simulink model "SwitchedPowerRelay_harness"  (Simulink 7.7)
settings: Solver=FixedStepDiscrete  SolverMode=SingleTasking  StartTime=0.0  StopTime=100  FixedStep=srate  RelTol=1e-3
InitFcn:
  | if signalbuilder('SwitchedPowerRelay_harness/Signal_Builder','activegroup') == 7
  |   CD_SWITCHED_POWER_RELAY_DEBOUNCE_NORMAL.DataType = 'uint16';
  |   CD_SWITCHED_POWER_RELAY_DEBOUNCE_NORMAL.Value = 65535;
  | else
  |   CD_SWITCHED_POWER_RELAY_DEBOUNCE_NORMAL.DataType = 'uint16';
  |   CD_SWITCHED_POWER_RELAY_DEBOUNCE_NORMAL.Value = 300;
  | end
  | 
  | if signalbuilder('SwitchedPowerRelay_harness/Signal_Builder','activegroup') == 1
  |   CD_SWITCHED_POWER_RELAY_FUNCTION.DataType = 'uint8';
  |   CD_SWITCHED_POWER_RELAY_FUNCTION.Value = 255;
  | else
  |   CD_SWITCHED_POWER_RELAY_FUNCTION.DataType = 'uint8';
  |   CD_SWITCHED_POWER_RELAY_FUNCTION.Value = 0;
  | end
  | 
  | if signalbuilder('SwitchedPowerRelay_harness/Signal_Builder','activegroup') == 2
  |   CD_SWITCHED_POWER_RELAY_FEEDBACK_FUNCTION.DataType = 'uint8';
  |   CD_SWITCHED_POWER_RELAY_FEEDBACK_FUNCTION.Value = 255;
  | else
  |   CD_SWITCHED_POWER_RELAY_FEEDBACK_FUNCTION.DataType = 'uint8';
  |   CD_SWITCHED_POWER_RELAY_FEEDBACK_FUNCTION.Value = 0;
  | end
undefined symbols (not defined in the file): ACTIVE, CD_SWITCHED_POWER_RELAY_DEBOUNCE_ERROR_ON, CD_SWITCHED_POWER_RELAY_DEBOUNCE_SHUTDOWN, INACTIVE, NON_FUNCTIONAL, OORL, sigbuilder_block, srate, SYS_LIMITED, SYS_POWER_DOWN
libraries: simulink x3, MX_Library x1
Description:
  | Determines state and error condition of the output.
CloseFcn:
  | rtwprivate ssgencode ModelCloseRequest sle_main_controller
settings Model: Creator=smindeman  LastModifiedBy=aliebel  ModifiedComment=smindema -- Wed Nov 01 14:11:02 2006 -- Version 1.321  CovPath=/SLE_Main  CovMetricSettings=dcm  CovHTMLOptions=-aTS=1 -bRG=1 -bTC=1 -hTR=0 -nFC=0 -scm=1 -bcm=1 -xEv=0  covSaveCumulativeToWorkspaceVar=off  CovSaveSingleToWorkspaceVar=off  CovModelRefEnable=off
settings Model: ModifiedHistory=|
  | smindema -- Wed Nov 01 14:11:02 2006 -- Version 1.321
  | 
  | 
  | smindema -- Wed Nov 01 14:09:50 2006 -- Version 1.320
  | added delay on startup to detect error on condition
  | 
  | smindema -- Wed Nov 01 14:09:44 2006 -- Version 1.319
  | 
  | 
  | smindema -- Fri Sep 29 09:20:06 2006 -- Version 1.318
  | updated based on build results
  | 
  | smindema -- Fri Sep 29 09:16:34 2006 -- Version 1.317
  | added open circuit detection
  | 
  | smindema -- Mon Aug 07 10:00:33 2006 -- Version 1.316
  | 
  | 
  | smindema -- Thu Aug 03 10:08:53 2006 -- Version 1.315
  |  removed initialization optimization
  | 
  | smindema -- Thu Jun 08 10:48:55 2006 -- Version 1.314
  | changed optimization settings
  | 
  | smindema -- Thu Apr 20 17:05:53 2006 -- Version 1.313
  | 
  | 
  | smindema -- Thu Apr 20 17:05:12 2006 -- Version 1.311
  | Changed so relay does not turn off with mulitple key.
  | 
  | smindema -- Thu Apr 20 17:05:12 2006 -- Version 1.311
  | Changed so relay does not turn off with mulitple key.
  | 
  | smindema -- Mon Mar 27 16:24:22 2006 -- Version 1.310
  | made dependent on light output.
  | 
  | smindema -- Mon Mar 27 16:13:31 2006 -- Version 1.309
  | 
  | 
  | smindema -- Thu Mar 09 15:09:10 2006 -- Version 1.308
  | made literal lenght max 50
  | 
  | smindema -- Thu Mar 09 14:11:03 2006 -- Version 1.307
  | 
  | 
  | smindema -- Thu Mar 02 09:10:11 2006 -- Version 1.306
  | Made constants mpt parameters.
settings MATStruct: SampleTime=0.01  Offset=0  Priority=[1.0]
settings DataIOCC: LimitDataPoints=off  SaveOutput=off  SaveTime=off
settings OptimizationCC: InlineParams=on  InlineInvariantSignals=on  ExpressionFolding=off  StateBitsets=on  DataBitsets=on  UseTempVars=on  InitFltsAndDblsToZero=on  NoFixptDivByZeroProtection=on  EfficientFloat2IntCast=on
settings DebuggingCC: SaveWithParameterizedLinksMsg=none  SignalResolutionControl=TryResolveAll  MultiTaskDSMMsg=warning  MultiTaskCondExecSysMsg=none  IntegerOverflowMsg=none  ModelReferenceCSMismatchMessage=warning
settings HardwareCC: ProdBitPerInt=16  ProdBitPerPointer=16  ProdIntDivRoundTo=Zero  ProdEndianess=BigEndian  ProdWordSize=16  ProdHWDeviceType=Motorola HC12
settings ModelReferenceCC: ModelReferenceNumInstancesAllowed=Single
settings RTWCC: SystemTargetFile=ert.tlc  GenCodeOnly=on  TemplateMakefile=ert_default_tmf  Description=Real-Time Workshop Embedded Coder (no auto configuration)  GenerateReport=on  RetainRTWFile=on  ProcessScript=ert_make_rtw_hook  IncludeHyperlinkInReport=on  LaunchReport=on  IncludeERTFirstTime=on
settings RTWCC: CustomHeaderCode=|
  | #include "cpp_req_defines.h"
  | #include "cdata.h"
settings CodeAppCC: IgnoreCustomStorageClasses=off  MaxIdLength=50  DefineNamingRule=UpperCase
settings ERTTargetCC: TargetFcnLib=ansi_tfl_tmw.mat  FunctionExecutionProfile=off  MultiwordLength=2048  GenerateSampleERTMain=on  IncludeMdlTerminateFcn=off  SuppressErrorStatus=on  SupportNonFinite=off  SupportComplex=off  PurelyIntegerCode=on  ERTCustomFileTemplate=gen_rtw_req_defines_h.tlc  GlobalDataDefinition=InSeparateSourceFile  GlobalDataReference=InSeparateHeaderFile  ConvertIfToSwitch=off

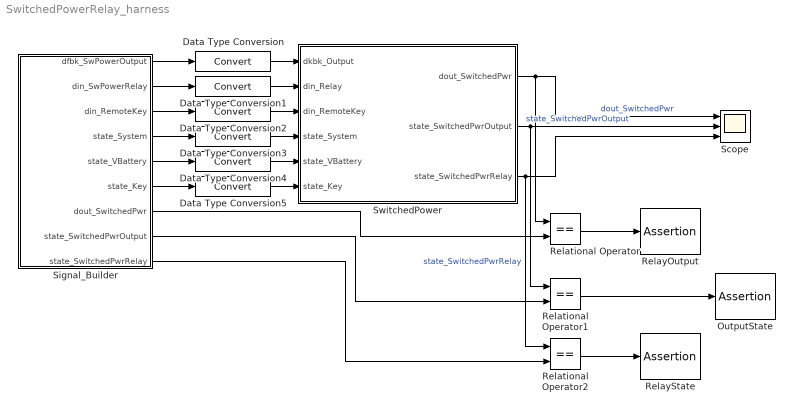
== system SwitchedPowerRelay_harness ==
  Data Type Conversion{,1..5} (6 alike) : DataTypeConversion
  OutputState : Assertion  Enabled=off
  Relational Operator : RelationalOperator  Operator===  OutDataTypeStr=boolean
  Relational Operator1 : RelationalOperator  Operator===  OutDataTypeStr=boolean
  Relational Operator2 : RelationalOperator  Operator===  OutDataTypeStr=boolean
  RelayOutput : Assertion  Enabled=off
  RelayState : Assertion  Enabled=off
  Scope : Scope  NumInputPorts=3
      settings: TimeRange=100  YMin=0~5~7  YMax=1~30~9  MaxDataPoints=50000
  Signal_Builder : Subsystem  Tag=STV Subsys  LoadFcn=sigbuilder_block('load');  StartFcn=sigbuilder_block('start');  StopFcn=sigbuilder_block('stop');  ClipboardFcn=sigbuilder_block('clipboard');  mask(Sigbuilder block){}
      mask help: Sigbuilder GUI
      mask init:
      | if ~strcmp(get_param(bdroot(gcbh),'SimulationStatus'),'stopped') tuvar = sigbuilder_block('maskInit'); end
      settings: CopyFcn=sigbuilder_block('copy');  DeleteFcn=sigbuilder_block('delete');  ModelCloseFcn=sigbuilder_block('modelClose');  PreSaveFcn=sigbuilder_block('preSave');  NameChangeFcn=sigbuilder_block('namechange');  OpenFcn=sigbuilder_block('open',[1510.5 183 1080 624.75 ]);  CloseFcn=sigbuilder_block('close');
      mask Display: plot(0,0,100,100,[10,10,40,40,10],[80,20,20,80,80],[40,10],[50,50], [40,27,10],[65,72,56],[40,25,25,10],[28,28,43,43]);
  SwitchedPower : Subsystem  TreatAsAtomicUnit=on  SystemSampleTime=srate  RTWFileName=mod_Outputs
      settings: RTWSystemCode=Function  RTWFileNameOpts=User specified
  wires:
  Relational Operator/1 -> RelayOutput/1
  Relational Operator1/1 -> OutputState/1
  Relational Operator2/1 -> RelayState/1
  SwitchedPower/1(dout_SwitchedPwr) -> Scope/1, Relational Operator/1  "dout_SwitchedPwr"
  SwitchedPower/2(state_SwitchedPwrOutput) -> Scope/2, Relational Operator1/1  "state_SwitchedPwrOutput"
  SwitchedPower/3(state_SwitchedPwrRelay) -> Scope/3, Relational Operator2/1  "state_SwitchedPwrRelay"
  Signal_Builder/1(dfbk_SwPowerOutput) -> Data Type Conversion/1
  Signal_Builder/2(din_SwPowerRelay) -> Data Type Conversion1/1
  Signal_Builder/3(din_RemoteKey) -> Data Type Conversion2/1
  Signal_Builder/4(state_System) -> Data Type Conversion3/1
  Signal_Builder/5(state_VBattery) -> Data Type Conversion4/1
  Signal_Builder/7(dout_SwitchedPwr) -> Relational Operator/2
  Signal_Builder/8(state_SwitchedPwrOutput) -> Relational Operator1/2
  Signal_Builder/9(state_SwitchedPwrRelay) -> Relational Operator2/2
  Data Type Conversion/1 -> SwitchedPower/1(dkbk_Output)
  Data Type Conversion1/1 -> SwitchedPower/2(din_Relay)
  Data Type Conversion2/1 -> SwitchedPower/3(din_RemoteKey)
  Data Type Conversion3/1 -> SwitchedPower/4(state_System)
  Data Type Conversion4/1 -> SwitchedPower/5(state_VBattery)
  Data Type Conversion5/1 -> SwitchedPower/6(state_Key)
  Signal_Builder/6(state_Key) -> Data Type Conversion5/1

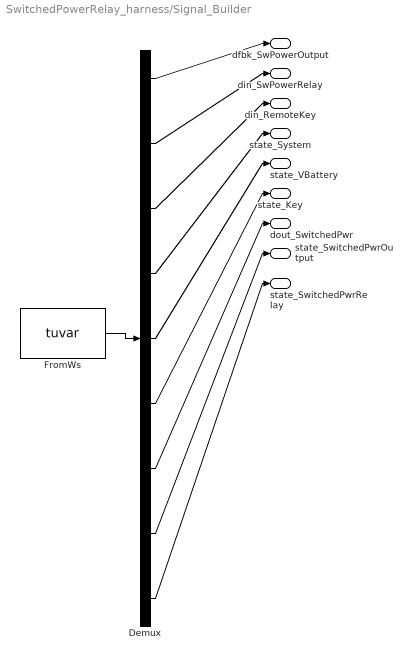
== system SwitchedPowerRelay_harness/Signal_Builder ==
  Demux : Demux  Tag=STV Demux  Outputs=9
  FromWs : FromWorkspace  Tag=STV FromWs  VariableName=tuvar  SampleTime=0  SigBuilderData=DataTag0  VnvData=DataTag1
      SigBuilderData=|
      | common.afterFinalStr = 'Extrapolate'
      | common.sampleTime = 0
      | dataSet(1).timeRange = [0 100]
      | dataSet(1).name = 'T1-Nonfunc'
      | dataSet(2).timeRange = [0 100]
      | dataSet(2).name = 'T2-No_feedback'
      | dataSet(3).timeRange = [0 100]
      | dataSet(3).name = 'T3-NORMAL'
      | dataSet(4).timeRange = [0 100]
      | dataSet(4).name = 'T4-OUT_ERROR'
      | dataSet(5).timeRange = [0 100]
      | dataSet(5).name = 'T5-RELAY_ERROR'
      | dataSet(6).timeRange = [0 100]
      | dataSet(6).name = 'T6-OC_FAILURE'
      | dataSet(7).timeRange = [0 100]
      | dataSet(7).name = 'T7-ERR_UNLIMITED'
      | sbobj.Groups(1).Name = 'T1-Nonfunc'
      | sbobj.Groups(1).Signals(1).Name = 'dfbk_SwPowerOutput'
      | sbobj.Groups(1).Signals(1).XData = [0 40.6 100]
      | sbobj.Groups(1).Signals(1).YData = [0 0 0]
      | sbobj.Groups(1).Signals(2).Name = 'din_SwPowerRelay'
      | sbobj.Groups(1).Signals(2).XData = [0 40.6 100]
      | sbobj.Groups(1).Signals(2).YData = [0 0 0]
      | sbobj.Groups(1).Signals(3).Name = 'din_RemoteKey'
      | sbobj.Groups(1).Signals(3).XData = [0 100]
      | sbobj.Groups(1).Signals(3).YData = [8 8]
      | sbobj.Groups(1).Signals(4).Name = 'state_System'
      | sbobj.Groups(1).Signals(4).XData = [0 40 40 100]
      | sbobj.Groups(1).Signals(4).YData = [0 0 1 1]
      | sbobj.Groups(1).Signals(5).Name = 'state_VBattery'
      | sbobj.Groups(1).Signals(5).XData = [0 100]
      | sbobj.Groups(1).Signals(5).YData = [8 8]
      | sbobj.Groups(1).Signals(6).Name = 'state_Key'
      | sbobj.Groups(1).Signals(6).XData = [0 100]
      | sbobj.Groups(1).Signals(6).YData = [0 0]
      | sbobj.Groups(1).Signals(7).Name = 'dout_SwitchedPwr'
      | sbobj.Groups(1).Signals(7).XData = [0 40.6 100]
      | sbobj.Groups(1).Signals(7).YData = [0 0 0]
      | sbobj.Groups(1).Signals(8).Name = 'state_SwitchedPwrOutput'
      | sbobj.Groups(1).Signals(8).XData = [0 100]
      | sbobj.Groups(1).Signals(8).YData = [8 8]
      | sbobj.Groups(1).Signals(9).Name = 'state_SwitchedPwrRelay'
      | sbobj.Groups(1).Signals(9).XData = [0 100]
      | sbobj.Groups(1).Signals(9).YData = [8 8]
      | sbobj.Groups(2).Name = 'T2-No_feedback'
      | sbobj.Groups(2).Signals(1).Name = 'dfbk_SwPowerOutput'
      | sbobj.Groups(2).Signals(1).XData = [0 40.6 100]
      | sbobj.Groups(2).Signals(1).YData = [0 0 0]
      | sbobj.Groups(2).Signals(2).Name = 'din_SwPowerRelay'
      | sbobj.Groups(2).Signals(2).XData = [0 40.6 100]
      | sbobj.Groups(2).Signals(2).YData = [0 0 0]
      | sbobj.Groups(2).Signals(3).Name = 'din_RemoteKey'
      | sbobj.Groups(2).Signals(3).XData = [0 100]
      | sbobj.Groups(2).Signals(3).YData = [0 0]
      | sbobj.Groups(2).Signals(4).Name = 'state_System'
      | sbobj.Groups(2).Signals(4).XData = [0 10 10 100]
      | sbobj.Groups(2).Signals(4).YData = [0 0 1 1]
      | sbobj.Groups(2).Signals(5).Name = 'state_VBattery'
      | sbobj.Groups(2).Signals(5).XData = [0 62.3 62.3 64.8 64.8 100]
      | sbobj.Groups(2).Signals(5).YData = [8 8 22 22 8 8]
      | sbobj.Groups(2).Signals(6).Name = 'state_Key'
      | sbobj.Groups(2).Signals(6).XData = [0 40.4 40.4 100]
      | sbobj.Groups(2).Signals(6).YData = [0 0 1 1]
      | sbobj.Groups(2).Signals(7).Name = 'dout_SwitchedPwr'
      | sbobj.Groups(2).Signals(7).XData = [0 40.46 40.46 100]
      | sbobj.Groups(2).Signals(7).YData = [0 0 1 1]
      | sbobj.Groups(2).Signals(8).Name = 'state_SwitchedPwrOutput'
      | sbobj.Groups(2).Signals(8).XData = [0 100]
      | sbobj.Groups(2).Signals(8).YData = [8 8]
      | sbobj.Groups(2).Signals(9).Name = 'state_SwitchedPwrRelay'
      | sbobj.Groups(2).Signals(9).XData = [0 100]
      | sbobj.Groups(2).Signals(9).YData = [8 8]
      | sbobj.Groups(3).Name = 'T3-NORMAL'
      | sbobj.Groups(3).Signals(1).Name = 'dfbk_SwPowerOutput'
      | sbobj.Groups(3).Signals(1).XData = [0 10.06 10.06 20 20 30 30 40 40 50 50 60 60 70.06 70.06 75.21 75.21 100]
      | sbobj.Groups(3).Signals(1).YData = [0 0 1 1 0 0 1 1 0 0 1 1 0 0 1 1 0 0]
      | sbobj.Groups(3).Signals(2).Name = 'din_SwPowerRelay'
      | sbobj.Groups(3).Signals(2).XData = [0 10.07 10.07 20 20 30 30 40 40 50 50 60 60 70.07 70.07 75.22 75.22 100]
      | sbobj.Groups(3).Signals(2).YData = [0 0 1 1 0 0 1 1 0 0 1 1 0 0 1 1 0 0]
      | sbobj.Groups(3).Signals(3).Name = 'din_RemoteKey'
      | sbobj.Groups(3).Signals(3).XData = [0 30 30 40 40 50 50 60 60 66.1 66.1 67.3 67.3 100]
      | sbobj.Groups(3).Signals(3).YData = [0 0 1 1 0 0 1 1 0 0 1 1 0 0]
      | sbobj.Groups(3).Signals(4).Name = 'state_System'
      | sbobj.Groups(3).Signals(4).XData = [0 10.7 10.7 20 20 21.5 21.5 30.5 30.5 40 40 41.4 41.4 50.4 50.4 60 60 68.6 68.6 75 75 78.7 78.7 100]
      | sbobj.Groups(3).Signals(4).YData = [0 0 1 1 5 5 0 0 1 1 5 5 0 0 1 1 5 5 0 0 3 3 0 0]
      | sbobj.Groups(3).Signals(5).Name = 'state_VBattery'
      | sbobj.Groups(3).Signals(5).XData = [0 100]
      | sbobj.Groups(3).Signals(5).YData = [8 8]
      | sbobj.Groups(3).Signals(6).Name = 'state_Key'
      | sbobj.Groups(3).Signals(6).XData = [0 10 10 20 20 50 50 60 60 64.3 64.3 65.1 65.1 70 70 75.01 75.01 100]
      | sbobj.Groups(3).Signals(6).YData = [0 0 1 1 0 0 1 1 0 0 1 1 0 0 1 1 0 0]
      | sbobj.Groups(3).Signals(7).Name = 'dout_SwitchedPwr'
      | sbobj.Groups(3).Signals(7).XData = [0 10.05 10.05 20.21 20.21 30 30 40.21 40.21 50 50 60.21 60.21 70.05 70.05 75.22 75.22 100]
      | sbobj.Groups(3).Signals(7).YData = [0 0 1 1 0 0 1 1 0 0 1 1 0 0 1 1 0 0]
      | sbobj.Groups(3).Signals(8).Name = 'state_SwitchedPwrOutput'
      | sbobj.Groups(3).Signals(8).XData = [0 100]
      | sbobj.Groups(3).Signals(8).YData = [8 8]
      | sbobj.Groups(3).Signals(9).Name = 'state_SwitchedPwrRelay'
      | sbobj.Groups(3).Signals(9).XData = [0 100]
      | sbobj.Groups(3).Signals(9).YData = [8 8]
      | sbobj.Groups(4).Name = 'T4-OUT_ERROR'
      | sbobj.Groups(4).Signals(1).Name = 'dfbk_SwPowerOutput'
      | sbobj.Groups(4).Signals(1).XData = [0 5.6 19.8 22.8 30 30 30.03 30.03 41.6 41.6 45 45 45.02 45.02 50.1 50.1 50.22 50.22 58.7 58.7 58.9 58.9 84.3 84.3 85 85 100]
      | sbobj.Groups(4).Signals(1).YData = [1 1 1 1 1 0 0 1 1 0 0 1 1 0 0 1 1 0 0 1 1 0 0 1 1 0 0]
      | sbobj.Groups(4).Signals(2).Name = 'din_SwPowerRelay'
      | sbobj.Groups(4).Signals(2).XData = [0 13.5 13.5 13.51 13.51 30 30 30.03 30.03 41.6 41.6 45 45 45.02 45.02 100]
      | sbobj.Groups(4).Signals(2).YData = [1 1 0 0 1 1 0 0 1 1 0 0 1 1 0 0]
      | sbobj.Groups(4).Signals(3).Name = 'din_RemoteKey'
      | sbobj.Groups(4).Signals(3).XData = [0 50 50 70.1 70.1 100]
      | sbobj.Groups(4).Signals(3).YData = [0 0 1 1 0 0]
      | sbobj.Groups(4).Signals(4).Name = 'state_System'
      | sbobj.Groups(4).Signals(4).XData = [0 20.4 20.4 40 40 41.6 41.6 50 50 70.1 70.1 72.3 72.3 84.3 84.3 84.8 84.8 100]
      | sbobj.Groups(4).Signals(4).YData = [0 0 1 1 5 5 0 0 1 1 5 5 0 0 3 3 0 0]
      | sbobj.Groups(4).Signals(5).Name = 'state_VBattery'
      | sbobj.Groups(4).Signals(5).XData = [0 100]
      | sbobj.Groups(4).Signals(5).YData = [8 8]
      | sbobj.Groups(4).Signals(6).Name = 'state_Key'
      | sbobj.Groups(4).Signals(6).XData = [0 20 20 40 40 80.1 80.1 81.4 81.4 100]
      | sbobj.Groups(4).Signals(6).YData = [0 0 1 1 0 0 1 1 0 0]
      | sbobj.Groups(4).Signals(7).Name = 'dout_SwitchedPwr'
      | sbobj.Groups(4).Signals(7).XData = [0 20.05 20.05 40.21 40.21 50 50 70.31 70.31 80.15 80.15 84.52 84.52 100]
      | sbobj.Groups(4).Signals(7).YData = [0 0 1 1 0 0 1 1 0 0 1 1 0 0]
      | sbobj.Groups(4).Signals(8).Name = 'state_SwitchedPwrOutput'
      | sbobj.Groups(4).Signals(8).XData = [0 0.04 0.04 23.06 23.06 50.53 50.53 70.1 70.1 80.46 80.46 84.83 84.83 88.01 88.01 100]
      | sbobj.Groups(4).Signals(8).YData = [8 8 2 2 8 8 3 3 8 8 3 3 7 7 8 8]
      | sbobj.Groups(4).Signals(9).Name = 'state_SwitchedPwrRelay'
      | sbobj.Groups(4).Signals(9).XData = [0 100]
      | sbobj.Groups(4).Signals(9).YData = [8 8]
      | sbobj.Groups(5).Name = 'T5-RELAY_ERROR'
      | sbobj.Groups(5).Signals(1).Name = 'dfbk_SwPowerOutput'
      | sbobj.Groups(5).Signals(1).XData = [0 5.5 5.5 5.52 5.52 10.7 10.7 21.9 21.9 22.1 22.1 42.7 42.7 44 44.01 50 50 62.1 62.1 62.2 62.2 91 91 100]
      | sbobj.Groups(5).Signals(1).YData = [0 0 1 1 0 0 1 1 0 0 1 1 0 0 0 0 0.98 0.98 0 0 0.98 0.98 0 0]
      | sbobj.Groups(5).Signals(2).Name = 'din_SwPowerRelay'
      | sbobj.Groups(5).Signals(2).XData = [0 42.8 42.8 45 45 45.01 45.01 100]
      | sbobj.Groups(5).Signals(2).YData = [1 1 0 0 1 1 0 0]
      | sbobj.Groups(5).Signals(3).Name = 'din_RemoteKey'
      | sbobj.Groups(5).Signals(3).XData = [0 50 50 90.9 90.9 100]
      | sbobj.Groups(5).Signals(3).YData = [0 0 1 1 0 0]
      | sbobj.Groups(5).Signals(4).Name = 'state_System'
      | sbobj.Groups(5).Signals(4).XData = [0 10 10 42 42 43.7 43.7 50 50 91.7 91.7 94.5 94.5 100]
      | sbobj.Groups(5).Signals(4).YData = [0 0 1 1 5 5 0 0 1 1 5 5 0 0]
      | sbobj.Groups(5).Signals(5).Name = 'state_VBattery'
      | sbobj.Groups(5).Signals(5).XData = [0 100]
      | sbobj.Groups(5).Signals(5).YData = [8 8]
      | sbobj.Groups(5).Signals(6).Name = 'state_Key'
      | sbobj.Groups(5).Signals(6).XData = [0 10 10 41.5 41.5 100]
      | sbobj.Groups(5).Signals(6).YData = [0 0 1 1 0 0]
      | sbobj.Groups(5).Signals(7).Name = 'dout_SwitchedPwr'
      | sbobj.Groups(5).Signals(7).XData = [0 10.05 10.05 42.21 42.21 50 50 91.91 91.91 100]
      | sbobj.Groups(5).Signals(7).YData = [0 0 1 1 0 0 1 1 0 0]
      | sbobj.Groups(5).Signals(8).Name = 'state_SwitchedPwrOutput'
      | sbobj.Groups(5).Signals(8).XData = [0 100]
      | sbobj.Groups(5).Signals(8).YData = [8 8]
      | sbobj.Groups(5).Signals(9).Name = 'state_SwitchedPwrRelay'
      | sbobj.Groups(5).Signals(9).XData = [0 0.04 0.04 13.06 13.06 50.31 50.31 91.7 91.7 100]
      | sbobj.Groups(5).Signals(9).YData = [8 8 2 2 8 8 3 3 8 8]
      | sbobj.Groups(6).Name = 'T6-OC_FAILURE'
      | sbobj.Groups(6).Signals(1).Name = 'dfbk_SwPowerOutput'
      | sbobj.Groups(6).Signals(1).XData = [0 1.03 1.03 1.06 1.06 14 14 14.05 14.05 40 40 50.1 50.1 50.2 50.2 50.3 50.3 54.9 54.9 62.8 62.8 100]
      | sbobj.Groups(6).Signals(1).YData = [0 0 1 1 0 0 1 1 0 0 1 1 0 0 1 1 0 0 1 1 0 0]
      | sbobj.Groups(6).Signals(2).Name = 'din_SwPowerRelay'
      | sbobj.Groups(6).Signals(2).XData = [0 1.03 1.03 18.1 18.1 18.15 18.15 19.9 19.9 55.08 55.08 57.43 57.43 61 61 61.7 61.7 100]
      | sbobj.Groups(6).Signals(2).YData = [0 0 1 1 0 0 1 1 0 0 1 1 0 0 1 1 0 0]
      | sbobj.Groups(6).Signals(3).Name = 'din_RemoteKey'
      | sbobj.Groups(6).Signals(3).XData = [0 100]
      | sbobj.Groups(6).Signals(3).YData = [0 0]
      | sbobj.Groups(6).Signals(4).Name = 'state_System'
      | sbobj.Groups(6).Signals(4).XData = [0 1.5 1.5 19.9 19.9 22.1 22.1 57.2 57.2 58.6 58.6 100]
      | sbobj.Groups(6).Signals(4).YData = [0 0 1 1 5 5 0 0 5 5 0 0]
      | sbobj.Groups(6).Signals(5).Name = 'state_VBattery'
      | sbobj.Groups(6).Signals(5).XData = [0 100]
      | sbobj.Groups(6).Signals(5).YData = [8 8]
      | sbobj.Groups(6).Signals(6).Name = 'state_Key'
      | sbobj.Groups(6).Signals(6).XData = [0 1 1 20 20 55 55 57.2 57.2 100]
      | sbobj.Groups(6).Signals(6).YData = [0 0 1 1 0 0 1 1 0 0]
      | sbobj.Groups(6).Signals(7).Name = 'dout_SwitchedPwr'
      | sbobj.Groups(6).Signals(7).XData = [0 1.05 1.05 20.11 20.11 55.05 55.05 57.41 57.41 100]
      | sbobj.Groups(6).Signals(7).YData = [0 0 1 1 0 0 1 1 0 0]
      | sbobj.Groups(6).Signals(8).Name = 'state_SwitchedPwrOutput'
      | sbobj.Groups(6).Signals(8).XData = [0 1.37 1.37 19.9 19.9 40.31 40.31 53.31 53.31 58.91 58.91 61.04 61.04 62.02 62.02 65.81 65.81 100]
      | sbobj.Groups(6).Signals(8).YData = [8 8 28 28 8 8 7 7 8 8 7 7 2 2 7 7 8 8]
      | sbobj.Groups(6).Signals(9).Name = 'state_SwitchedPwrRelay'
      | sbobj.Groups(6).Signals(9).XData = [0 100]
      | sbobj.Groups(6).Signals(9).YData = [8 8]
      | sbobj.Groups(7).Name = 'T7-ERR_UNLIMITED'
      | sbobj.Groups(7).Signals(1).Name = 'dfbk_SwPowerOutput'
      | sbobj.Groups(7).Signals(1).XData = [0 5.6 41.6 41.6 50.1 50.1 50.13 50.13 56.9 56.9 57 57 75 75 75.02 75.02 76 76 78.4 78.4 100]
      | sbobj.Groups(7).Signals(1).YData = [1 1 1 0 0 1 1 0 0 1 1 0 0 1 1 0 0 1 1 0 0]
      | sbobj.Groups(7).Signals(2).Name = 'din_SwPowerRelay'
      | sbobj.Groups(7).Signals(2).XData = [0 41.6 41.6 80.07 80.07 80.2 80.2 84.05 84.05 86.5 86.5 100]
      | sbobj.Groups(7).Signals(2).YData = [1 1 0 0 1 1 0 0 1 1 0 0]
      | sbobj.Groups(7).Signals(3).Name = 'din_RemoteKey'
      | sbobj.Groups(7).Signals(3).XData = [0 50 50 70.1 70.1 80.1 81.8 100]
      | sbobj.Groups(7).Signals(3).YData = [0 0 1 1 0 0 0 0]
      | sbobj.Groups(7).Signals(4).Name = 'state_System'
      | sbobj.Groups(7).Signals(4).XData = [0 20.4 20.4 40 40 41.6 41.6 50 50 70.1 70.1 72.3 72.3 79.4 79.4 79.7 79.7 80.1 80.1 80.2 80.2 88.6 88.6 90.3 90.3 100]
      | sbobj.Groups(7).Signals(4).YData = [0 0 1 1 5 5 0 0 1 1 5 5 0 0 5 5 0 0 3 3 0 0 5 5 0 0]
      | sbobj.Groups(7).Signals(5).Name = 'state_VBattery'
      | sbobj.Groups(7).Signals(5).XData = [0 97.7 97.7 98.5 98.5 100]
      | sbobj.Groups(7).Signals(5).YData = [8 8 22 22 8 8]
      | sbobj.Groups(7).Signals(6).Name = 'state_Key'
      | sbobj.Groups(7).Signals(6).XData = [0 20 20 40 40 80 80 80.1 80.1 84 84 86.9 86.9 100]
      | sbobj.Groups(7).Signals(6).YData = [0 0 1 1 0 0 1 1 0 0 1 1 0 0]
      | sbobj.Groups(7).Signals(7).Name = 'dout_SwitchedPwr'
      | sbobj.Groups(7).Signals(7).XData = [0 20.05 20.05 40.21 40.21 50 50 70.31 70.31 80.05 80.05 80.12 80.31 80.31 84.05 84.05 88.81 88.81 100]
      | sbobj.Groups(7).Signals(7).YData = [0 0 1 1 0 0 1 1 0 0 1 1 1 0 0 1 1 0 0]
      | sbobj.Groups(7).Signals(8).Name = 'state_SwitchedPwrOutput'
      | sbobj.Groups(7).Signals(8).XData = [0 0.04 0.04 40 40 50.44 50.44 70.1 70.1 76.31 76.31 79.4 79.4 84.36 84.36 88.6 88.6 100]
      | sbobj.Groups(7).Signals(8).YData = [8 8 2 2 8 8 3 3 8 8 7 7 8 8 28 28 8 8]
      | sbobj.Groups(7).Signals(9).Name = 'state_SwitchedPwrRelay'
      | sbobj.Groups(7).Signals(9).XData = [0 86.81 86.81 88.6 88.6 100]
      | sbobj.Groups(7).Signals(9).YData = [8 8 3 3 8 8]
  dfbk_SwPowerOutput : Outport  Tag=STV Outport
  din_SwPowerRelay : Outport  Tag=STV Outport  Port=2
  din_RemoteKey : Outport  Tag=STV Outport  Port=3
  state_System : Outport  Tag=STV Outport  Port=4
  state_VBattery : Outport  Tag=STV Outport  Port=5
  state_Key : Outport  Tag=STV Outport  Port=6
  dout_SwitchedPwr : Outport  Tag=STV Outport  Port=7
  state_SwitchedPwrOutput : Outport  Tag=STV Outport  Port=8
  state_SwitchedPwrRelay : Outport  Tag=STV Outport  Port=9
  wires:
  FromWs/1 -> Demux/1
  Demux/1 -> dfbk_SwPowerOutput/1
  Demux/2 -> din_SwPowerRelay/1
  Demux/3 -> din_RemoteKey/1
  Demux/4 -> state_System/1
  Demux/5 -> state_VBattery/1
  Demux/6 -> state_Key/1
  Demux/7 -> dout_SwitchedPwr/1
  Demux/8 -> state_SwitchedPwrOutput/1
  Demux/9 -> state_SwitchedPwrRelay/1

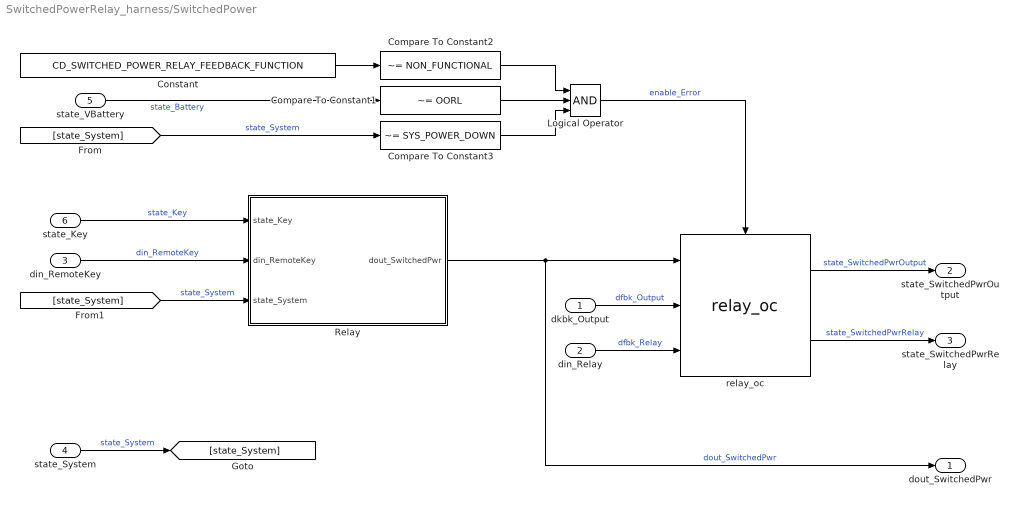
== system SwitchedPowerRelay_harness/SwitchedPower ==
  dkbk_Output : Inport
  din_Relay : Inport  Port=2
  din_RemoteKey : Inport  Port=3
  state_System : Inport  Port=4
  state_VBattery : Inport  Port=5
  state_Key : Inport  Port=6
  Compare To Constant1 : simulink/Logic and Bit Operations/Compare To Constant  SystemSampleTime=-1  relop=~=  const=OORL  LogicOutDataTypeMode=boolean  ZeroCross=off
  Compare To Constant2 : simulink/Logic and Bit Operations/Compare To Constant  SystemSampleTime=-1  relop=~=  const=NON_FUNCTIONAL  LogicOutDataTypeMode=boolean  ZeroCross=off
  Compare To Constant3 : simulink/Logic and Bit Operations/Compare To Constant  SystemSampleTime=-1  relop=~=  const=SYS_POWER_DOWN  LogicOutDataTypeMode=boolean  ZeroCross=off
  Constant : Constant  Value=CD_SWITCHED_POWER_RELAY_FEEDBACK_FUNCTION  OutDataTypeStr=uint8
  Logical Operator : Logic  Inputs=3  AllPortsSameDT=off  OutDataTypeStr=boolean
  Relay : Stateflow chart  TreatAsAtomicUnit=on
  relay_oc : MX_Library/relay_oc  SystemSampleTime=-1  ERROR_ON_DB_CNT=CD_SWITCHED_POWER_RELAY_DEBOUNCE_ERROR_ON  ERROR_OFF_DB_CNT=CD_SWITCHED_POWER_RELAY_DEBOUNCE_ERROR_OFF  NORMAL_DB_CNT=CD_SWITCHED_POWER_RELAY_DEBOUNCE_NORMAL
  dout_SwitchedPwr : Outport
  state_SwitchedPwrOutput : Outport  Port=2
  state_SwitchedPwrRelay : Outport  Port=3
  wires:
  state_Key/1 -> Relay/1(state_Key)  "state_Key"
  din_RemoteKey/1 -> Relay/2(din_RemoteKey)  "din_RemoteKey"
  Relay/1(dout_SwitchedPwr) -> relay_oc/1, dout_SwitchedPwr/1  "dout_SwitchedPwr"
  Constant/1 -> Compare To Constant2/1
  Compare To Constant2/1 -> Logical Operator/1
  Logical Operator/1 -> relay_oc/Enable  "enable_Error"
  Compare To Constant1/1 -> Logical Operator/2
  state_VBattery/1 -> Compare To Constant1/1  "state_Battery"
  relay_oc/1 -> state_SwitchedPwrOutput/1  "state_SwitchedPwrOutput"
  relay_oc/2 -> state_SwitchedPwrRelay/1  "state_SwitchedPwrRelay"
  dkbk_Output/1 -> relay_oc/2  "dfbk_Output"
  din_Relay/1 -> relay_oc/3  "dfbk_Relay"
  [state_System] -> Compare To Constant3/1  "state_System"
  Compare To Constant3/1 -> Logical Operator/3
  state_System/1 -> [state_System]  "state_System"
  [state_System] -> Relay/3(state_System)  "state_System"

== stateflow chart SwitchedPower/Relay ==
  state INACTIVE
    en:dout_SwitchedPwr = INACTIVE;
  state ACTIVE
    en:dout_SwitchedPwr = ACTIVE;
  state DEBOUNCE_ERROR_ON_CHECK
    en:debounceCount = 0;
    du:debounceCount++;
  note: Delay switched power relay for a short period of time
      | to allow error detection.  Do not delay if turned on with
      | service tool.  Suitcase service tool turns on switched power
      | which causes a false alarm.
  state DELAY_OFF
    en:debounceCount = 0;
    du:debounceCount++;
  note: Delay shutdown to give enough time for
      | shutdown message to be sent out so
      | you don't get nuicanse joystick alarms.
  (default) -> INACTIVE
  INACTIVE -> DEBOUNCE_ERROR_ON_CHECK [order 1] : [(state_Key != INACTIVE)...
      | && (din_RemoteKey == INACTIVE)...
      | && (state_System != SYS_POWER_DOWN)]
  ACTIVE -> DELAY_OFF : [(state_System == SYS_POWER_DOWN)...
      | || ((state_System == SYS_LIMITED) && (state_Key == INACTIVE))]
  DEBOUNCE_ERROR_ON_CHECK -> ACTIVE : [(debounceCount >= (CD_SWITCHED_POWER_RELAY_DEBOUNCE_ERROR_ON + 2))]
  INACTIVE -> ACTIVE [order 2] : [(din_RemoteKey == ACTIVE)...
      | && (state_System != SYS_POWER_DOWN)]
  DELAY_OFF -> INACTIVE : [(debounceCount >= CD_SWITCHED_POWER_RELAY_DEBOUNCE_SHUTDOWN)]
  data: state_Key input uint8; dout_SwitchedPwr output boolean; INACTIVE parameter uint8; debounceCount local uint16; CD_SWITCHED_POWER_RELAY_DEBOUNCE_ERROR_ON parameter uint16; din_RemoteKey input uint8; CD_SWITCHED_POWER_RELAY_DEBOUNCE_SHUTDOWN parameter uint16; ACTIVE parameter uint8; state_System input uint8; SYS_POWER_DOWN parameter uint8; SYS_LIMITED parameter uint8
